simulink model "PMSM_Trapezoidal_ToolBoxST"  (R2013b)
settings: Solver=FixedStepDiscrete  StartTime=0.0  StopTime=10.0  FixedStep=1/5000  RelTol=1e-3
libraries: GPIO_Lib x7, ADC_Lib x3, simulink x3, TIMERS_Lib x1
settings Model: SimulationMode=accelerator  Creator=Alex  LastModifiedBy=reynaudp
settings OptimizationCC: ExpressionDepthLimit=2147483647  OptimizeModelRefInitCode=on  LifeSpan=1
settings DebuggingCC: StateNameClashWarn=warning
settings HardwareCC: ProdLargestAtomicInteger=Integer  ProdLargestAtomicFloat=Float  ProdIntDivRoundTo=Zero  ProdEndianess=LittleEndian  ProdHWDeviceType=STMicroelectronics->STM32F4xx 32-bit Cortex-M4  TargetLargestAtomicInteger=Integer  TargetLargestAtomicFloat=Float  TargetIntDivRoundTo=Zero  TargetEndianess=LittleEndian  TargetHWDeviceType=STMicroelectronics->STM32F4xx 32-bit Cortex-M4
settings RTWCC: SystemTargetFile=stm32F4xx.tlc  TemplateMakefile=stm32F4xx.tmf  Description=stm32F4xx (Embedded Target)  GenerateReport=on  ProcessScript=stm32F4xx_make_rtw_hook  IncludeHyperlinkInReport=on  LaunchReport=on
settings CodeAppCC: IgnoreCustomStorageClasses=off  MaxIdLength=63  CustomSymbolStrType=$N$R$M  InternalIdentifier=Classic
settings STFCustomTargetCC: ParMdlRefBuildCompliant=on  IncludeMdlTerminateFcn=off  CombineOutputUpdateFcns=on  ERTCustomFileBanners=on  SupportContinuousTime=off  SupportNonInlinedSFcns=off  MATLABClassNameForMDSCustomization=Simulink.SoftwareTarget.ERTCustomization  GRTInterface=off  SystemTargetFile=stm32F4xx.tlc
settings ERTTargetCC: CodeReplacementLibrary=ANSI_C  CompOptLevelCompliant=off  ConcurrentExecutionCompliant=off  IncludeMdlTerminateFcn=off  ERTFirstTimeCompliant=off  ModelStepFunctionPrototypeControlCompliant=off  CPPClassGenCompliant=off  InlinedParameterPlacement=NonHierarchical  ERTSrcFileBannerTemplate=sourceFileTemplate.cgt  ERTHdrFileBannerTemplate=sourceFileTemplate.cgt  ERTDataSrcFileTemplate=sourceFileTemplate.cgt  ERTDataHdrFileTemplate=sourceFileTemplate.cgt  ERTCustomFileTemplate=customRoutineProcess.tlc

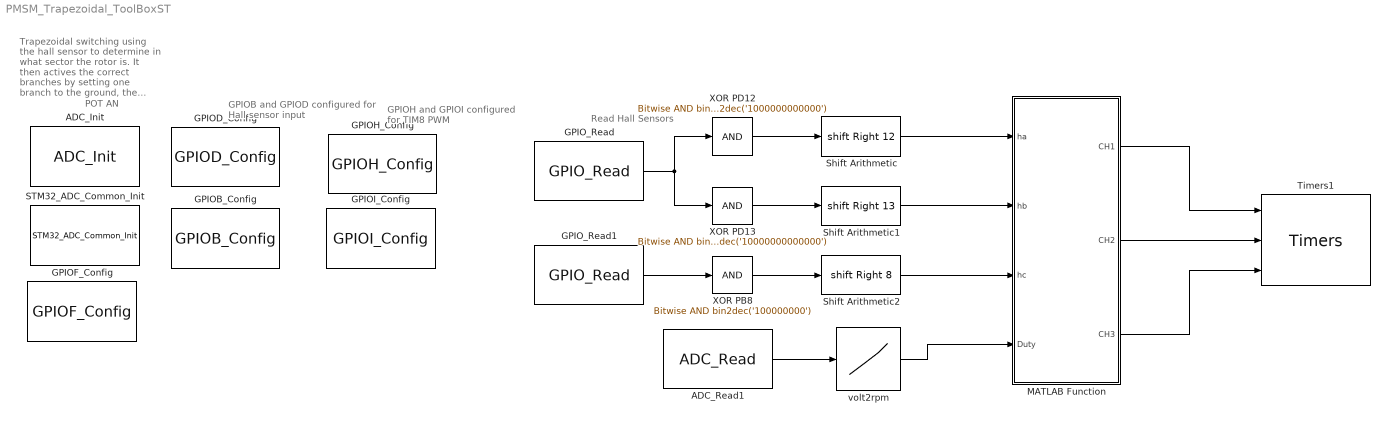
== system PMSM_Trapezoidal_ToolBoxST ==
  note: Trapezoidal switching using the hall sensor to determine in what sector the rotor is. It then actives the correct branches by setting one branch to the ground, the other floating, and the third as PWM pulsing.
      |
      | The PWM duty ratio determines the effective voltage, and thus the speed of the motor. The hall sensors are read using the GPIO, and then the duty is applied to the corresponding PWM channels according to a truth table.
      |
      | Using trapezoidal switching, the current vector is controlled at 30 degree intervals, meaning that the vector is NOT always at 90 degrees with the rotor (which is the optimal control method), but rather oscillates with an error of +- 30 degrees. In this case, a ripple in the torque applied, and the motor produces extra noise, and consumes more current for the same mechanical power output (loss of efficiency)
      |
      | This Algorithm works in open loop (The motor speed is not measured)
  note: POT AN
  note: Read Hall Sensors
  note: GPIOB and GPIOD
      | configured for Hall sensor input
  note: GPIOH and GPIOI
      | configured for TIM8 PWM
  ADC_Init : ADC_Lib/ADC_Init  ADC_Name=ADC3  ADC_Type=Regular  ADC_Default=off  ADC_Offset=0  ADC_Resolution=ADC_Resolution_12b  ADC_ScanConvMode=One_channel  ADC_ContinuousConvMode=on  ADC_ExtTrigPol=ADC_ExternalTrigConvEdge_None  ADC_ExtTrigInjPol=ADC_ExternalTrigInjecConvEdge_None  ADC_ExtTrig=ADC_ExternalTrigConv_T1_CC1  ADC_ExtTrigInj=ADC_ExternalTrigInjecConv_T1_CC4  ADC_DataAlign=ADC_DataAlign_Right  ADC_NbConv=1  ADC_DMA_channel=not_used  ADC_DMA_stream=not_used  ADC_Watchdog_Enable=off  ADC_Watchdog_Command=ADC_AnalogWatchdog_None  ADC_Watchdog_NumChan=0  ADC_Watchdog_HighThreshold=4095  ADC_Watchdog_lowThreshold=0  ADC_Ch0=off  ADC_Ch0T=Regular  ADC_Ch0L=PA0  ADC_Ch1=off  ADC_Ch1T=Regular  ADC_Ch1L=PA1  ADC_Ch2=off  ADC_Ch2T=Regular  ADC_Ch2L=PA2  ADC_Ch3=off  ADC_Ch3T=Regular  ADC_Ch3L=PA3  ADC_Ch4=off  ADC_Ch4T=Regular  ADC_Ch4L=PF6  ADC_Ch5=off  ADC_Ch5T=Regular  ADC_Ch5L=PF7  ADC_Ch6=off  ADC_Ch6T=Regular  ADC_Ch6L=PF8  ADC_Ch7=on  ADC_Ch7T=Regular  ADC_Ch7L=PF9  ADC_Ch8=off  ADC_Ch8T=Regular  ADC_Ch8L=PF10  ADC_Ch9=off  ADC_Ch9T=Regular  ADC_Ch9L=PF3  ADC_Ch10=off  ADC_Ch10T=Regular  ADC_Ch10L=PC0  ADC_Ch11=off  ADC_Ch11T=Regular  ADC_Ch11L=PC1  ADC_Ch12=off  ADC_Ch12T=Regular  ADC_Ch12L=PC2  ADC_Ch13=off  ADC_Ch13T=Regular  ADC_Ch13L=PC3  ADC_Ch14=off  ADC_Ch14T=Regular  ADC_Ch14L=PF4  ADC_Ch15=off  ADC_Ch15T=Regular  ADC_Ch15L=PF5  ADC_Ch16=off  ADC_Ch16T=Regular  ADC_Ch17=off  ADC_Ch17T=Regular  ADC_Ch18=off  ADC_Ch18T=Regular
  ADC_Read1 : ADC_Lib/ADC_Read  ADC_Name=ADC3  ADC_Ch0=off  ADC_Ch1=off  ADC_Ch2=off  ADC_Ch3=off  ADC_Ch4=off  ADC_Ch5=off  ADC_Ch6=off  ADC_Ch7=on  ADC_Ch8=off  ADC_Ch9=off  ADC_Ch10=off  ADC_Ch11=off  ADC_Ch12=off  ADC_Ch13=off  ADC_Ch14=off  ADC_Ch15=off  ADC_Ch16=off  ADC_Ch17=off  ADC_Ch18=off
  GPIOB_Config : GPIO_Lib/GPIOB_Config  Pin0_Use=off  Pin1_Use=off  Pin2_Use=off  Pin3_Use=off  Pin4_Use=off  Pin5_Use=off  Pin6_Use=off  Pin7_Use=off  Pin8_Use=on  Pin9_Use=off  Pin10_Use=off  Pin11_Use=off  Pin12_Use=off  Pin13_Use=off  Pin14_Use=off  Pin15_Use=off  Pin0_Speed=GPIO_Speed_2MHz  Pin1_Speed=GPIO_Speed_2MHz  Pin2_Speed=GPIO_Speed_2MHz  Pin3_Speed=GPIO_Speed_2MHz  Pin4_Speed=GPIO_Speed_2MHz  Pin5_Speed=GPIO_Speed_2MHz  Pin6_Speed=GPIO_Speed_2MHz  Pin7_Speed=GPIO_Speed_2MHz  Pin8_Speed=GPIO_Speed_50MHz  Pin9_Speed=GPIO_Speed_2MHz  Pin10_Speed=GPIO_Speed_2MHz  Pin11_Speed=GPIO_Speed_2MHz  Pin12_Speed=GPIO_Speed_2MHz  Pin13_Speed=GPIO_Speed_2MHz  Pin14_Speed=GPIO_Speed_2MHz  Pin15_Speed=GPIO_Speed_2MHz  Pin0_Mode=GPIO_Mode_OUT  Pin1_Mode=GPIO_Mode_OUT  Pin2_Mode=GPIO_Mode_OUT  Pin3_Mode=GPIO_Mode_OUT  Pin4_Mode=GPIO_Mode_OUT  Pin5_Mode=GPIO_Mode_OUT  Pin6_Mode=GPIO_Mode_OUT  Pin7_Mode=GPIO_Mode_OUT  Pin8_Mode=GPIO_Mode_IN  Pin9_Mode=GPIO_Mode_OUT  Pin10_Mode=GPIO_Mode_OUT  Pin11_Mode=GPIO_Mode_OUT  Pin12_Mode=GPIO_Mode_OUT  Pin13_Mode=GPIO_Mode_OUT  Pin14_Mode=GPIO_Mode_OUT  Pin15_Mode=GPIO_Mode_OUT  Pin0_Type=GPIO_OType_PP  Pin1_Type=GPIO_OType_PP  Pin2_Type=GPIO_OType_PP  Pin3_Type=GPIO_OType_PP  Pin4_Type=GPIO_OType_PP  Pin5_Type=GPIO_OType_PP  Pin6_Type=GPIO_OType_PP  Pin7_Type=GPIO_OType_PP  Pin8_Type=GPIO_OType_PP  Pin9_Type=GPIO_OType_PP  Pin10_Type=GPIO_OType_PP  Pin11_Type=GPIO_OType_PP  Pin12_Type=GPIO_OType_PP  Pin13_Type=GPIO_OType_PP  Pin14_Type=GPIO_OType_PP  Pin15_Type=GPIO_OType_PP  Pin0_PuPd=GPIO_PuPd_NOPULL  Pin1_PuPd=GPIO_PuPd_NOPULL  Pin2_PuPd=GPIO_PuPd_NOPULL  Pin3_PuPd=GPIO_PuPd_NOPULL  Pin4_PuPd=GPIO_PuPd_NOPULL  Pin5_PuPd=GPIO_PuPd_NOPULL  Pin6_PuPd=GPIO_PuPd_NOPULL  Pin7_PuPd=GPIO_PuPd_NOPULL  Pin8_PuPd=GPIO_PuPd_NOPULL  Pin9_PuPd=GPIO_PuPd_NOPULL  Pin10_PuPd=GPIO_PuPd_NOPULL  Pin11_PuPd=GPIO_PuPd_NOPULL  Pin12_PuPd=GPIO_PuPd_NOPULL  Pin13_PuPd=GPIO_PuPd_NOPULL  Pin14_PuPd=GPIO_PuPd_NOPULL  Pin15_PuPd=GPIO_PuPd_NOPULL  Pin0_AF=GPIO_AF_TIM1  Pin1_AF=GPIO_AF_TIM1  Pin3_AF=GPIO_AF_TIM2  Pin4_AF=GPIO_AF_SPI1  Pin5_AF=GPIO_AF_EVENTOUT  Pin6_AF=GPIO_AF_TIM4  Pin7_AF=GPIO_AF_TIM4  Pin8_AF=GPIO_AF_TIM4  Pin9_AF=GPIO_AF_TIM11  Pin10_AF=GPIO_AF_TIM2  Pin11_AF=GPIO_AF_TIM2  Pin12_AF=GPIO_AF_TIM1  Pin13_AF=GPIO_AF_TIM1  Pin14_AF=GPIO_AF_TIM1  Pin15_AF=GPIO_AF_EVENTOUT  Pin0_Set=off  Pin1_Set=off  Pin2_Set=off  Pin3_Set=off  Pin4_Set=off  Pin5_Set=off  Pin6_Set=off  Pin7_Set=off  Pin8_Set=off  Pin9_Set=off  Pin10_Set=off  Pin11_Set=off  Pin12_Set=off  Pin13_Set=off  Pin14_Set=off  Pin15_Set=off
  GPIOD_Config : GPIO_Lib/GPIOD_Config  Pin0_Use=off  Pin1_Use=off  Pin2_Use=off  Pin3_Use=off  Pin4_Use=off  Pin5_Use=off  Pin6_Use=off  Pin7_Use=off  Pin8_Use=off  Pin9_Use=off  Pin10_Use=off  Pin11_Use=off  Pin12_Use=on  Pin13_Use=on  Pin14_Use=off  Pin15_Use=off  Pin0_Speed=GPIO_Speed_2MHz  Pin1_Speed=GPIO_Speed_2MHz  Pin2_Speed=GPIO_Speed_2MHz  Pin3_Speed=GPIO_Speed_2MHz  Pin4_Speed=GPIO_Speed_2MHz  Pin5_Speed=GPIO_Speed_2MHz  Pin6_Speed=GPIO_Speed_2MHz  Pin7_Speed=GPIO_Speed_2MHz  Pin8_Speed=GPIO_Speed_2MHz  Pin9_Speed=GPIO_Speed_2MHz  Pin10_Speed=GPIO_Speed_2MHz  Pin11_Speed=GPIO_Speed_2MHz  Pin12_Speed=GPIO_Speed_100MHz  Pin13_Speed=GPIO_Speed_100MHz  Pin14_Speed=GPIO_Speed_2MHz  Pin15_Speed=GPIO_Speed_2MHz  Pin0_Mode=GPIO_Mode_OUT  Pin1_Mode=GPIO_Mode_OUT  Pin2_Mode=GPIO_Mode_OUT  Pin3_Mode=GPIO_Mode_OUT  Pin4_Mode=GPIO_Mode_OUT  Pin5_Mode=GPIO_Mode_OUT  Pin6_Mode=GPIO_Mode_OUT  Pin7_Mode=GPIO_Mode_OUT  Pin8_Mode=GPIO_Mode_OUT  Pin9_Mode=GPIO_Mode_OUT  Pin10_Mode=GPIO_Mode_OUT  Pin11_Mode=GPIO_Mode_OUT  Pin12_Mode=GPIO_Mode_IN  Pin13_Mode=GPIO_Mode_IN  Pin14_Mode=GPIO_Mode_OUT  Pin15_Mode=GPIO_Mode_OUT  Pin0_Type=GPIO_OType_PP  Pin1_Type=GPIO_OType_PP  Pin2_Type=GPIO_OType_PP  Pin3_Type=GPIO_OType_PP  Pin4_Type=GPIO_OType_PP  Pin5_Type=GPIO_OType_PP  Pin6_Type=GPIO_OType_PP  Pin7_Type=GPIO_OType_PP  Pin8_Type=GPIO_OType_PP  Pin9_Type=GPIO_OType_PP  Pin10_Type=GPIO_OType_PP  Pin11_Type=GPIO_OType_PP  Pin12_Type=GPIO_OType_PP  Pin13_Type=GPIO_OType_PP  Pin14_Type=GPIO_OType_PP  Pin15_Type=GPIO_OType_PP  Pin0_PuPd=GPIO_PuPd_NOPULL  Pin1_PuPd=GPIO_PuPd_NOPULL  Pin2_PuPd=GPIO_PuPd_NOPULL  Pin3_PuPd=GPIO_PuPd_NOPULL  Pin4_PuPd=GPIO_PuPd_NOPULL  Pin5_PuPd=GPIO_PuPd_NOPULL  Pin6_PuPd=GPIO_PuPd_NOPULL  Pin7_PuPd=GPIO_PuPd_NOPULL  Pin8_PuPd=GPIO_PuPd_NOPULL  Pin9_PuPd=GPIO_PuPd_NOPULL  Pin10_PuPd=GPIO_PuPd_NOPULL  Pin11_PuPd=GPIO_PuPd_NOPULL  Pin12_PuPd=GPIO_PuPd_NOPULL  Pin13_PuPd=GPIO_PuPd_NOPULL  Pin14_PuPd=GPIO_PuPd_NOPULL  Pin15_PuPd=GPIO_PuPd_NOPULL  Pin0_AF=GPIO_AF_CAN1  Pin1_AF=GPIO_AF_CAN1  Pin2_AF=GPIO_AF_TIM3  Pin3_AF=GPIO_AF_USART2  Pin4_AF=GPIO_AF_USART2  Pin5_AF=GPIO_AF_EVENTOUT  Pin6_AF=GPIO_AF_USART2  Pin7_AF=GPIO_AF_USART2  Pin8_AF=GPIO_AF_USART3  Pin9_AF=GPIO_AF_USART3  Pin10_AF=GPIO_AF_USART3  Pin11_AF=GPIO_AF_USART3  Pin12_AF=GPIO_AF_TIM4  Pin13_AF=GPIO_AF_TIM4  Pin14_AF=GPIO_AF_TIM4  Pin15_AF=GPIO_AF_EVENTOUT  Pin0_Set=off  Pin1_Set=off  Pin2_Set=off  Pin3_Set=off  Pin4_Set=off  Pin5_Set=off  Pin6_Set=off  Pin7_Set=off  Pin8_Set=off  Pin9_Set=off  Pin10_Set=off  Pin11_Set=off  Pin12_Set=off  Pin13_Set=off  Pin14_Set=off  Pin15_Set=off
  GPIOF_Config : GPIO_Lib/GPIOF_Config  Pin0_Use=off  Pin1_Use=off  Pin2_Use=off  Pin3_Use=off  Pin4_Use=off  Pin5_Use=off  Pin6_Use=off  Pin7_Use=off  Pin8_Use=off  Pin9_Use=on  Pin10_Use=off  Pin11_Use=off  Pin12_Use=off  Pin13_Use=off  Pin14_Use=off  Pin15_Use=off  Pin0_Speed=GPIO_Speed_2MHz  Pin1_Speed=GPIO_Speed_2MHz  Pin2_Speed=GPIO_Speed_2MHz  Pin3_Speed=GPIO_Speed_2MHz  Pin4_Speed=GPIO_Speed_2MHz  Pin5_Speed=GPIO_Speed_2MHz  Pin6_Speed=GPIO_Speed_2MHz  Pin7_Speed=GPIO_Speed_2MHz  Pin8_Speed=GPIO_Speed_2MHz  Pin9_Speed=GPIO_Speed_50MHz  Pin10_Speed=GPIO_Speed_2MHz  Pin11_Speed=GPIO_Speed_2MHz  Pin12_Speed=GPIO_Speed_2MHz  Pin13_Speed=GPIO_Speed_2MHz  Pin14_Speed=GPIO_Speed_2MHz  Pin15_Speed=GPIO_Speed_2MHz  Pin0_Mode=GPIO_Mode_OUT  Pin1_Mode=GPIO_Mode_OUT  Pin2_Mode=GPIO_Mode_OUT  Pin3_Mode=GPIO_Mode_OUT  Pin4_Mode=GPIO_Mode_OUT  Pin5_Mode=GPIO_Mode_OUT  Pin6_Mode=GPIO_Mode_OUT  Pin7_Mode=GPIO_Mode_OUT  Pin8_Mode=GPIO_Mode_OUT  Pin9_Mode=GPIO_Mode_AN  Pin10_Mode=GPIO_Mode_OUT  Pin11_Mode=GPIO_Mode_OUT  Pin12_Mode=GPIO_Mode_OUT  Pin13_Mode=GPIO_Mode_OUT  Pin14_Mode=GPIO_Mode_OUT  Pin15_Mode=GPIO_Mode_OUT  Pin0_Type=GPIO_OType_PP  Pin1_Type=GPIO_OType_PP  Pin2_Type=GPIO_OType_PP  Pin3_Type=GPIO_OType_PP  Pin4_Type=GPIO_OType_PP  Pin5_Type=GPIO_OType_PP  Pin6_Type=GPIO_OType_PP  Pin7_Type=GPIO_OType_PP  Pin8_Type=GPIO_OType_PP  Pin9_Type=GPIO_OType_PP  Pin10_Type=GPIO_OType_PP  Pin11_Type=GPIO_OType_PP  Pin12_Type=GPIO_OType_PP  Pin13_Type=GPIO_OType_PP  Pin14_Type=GPIO_OType_PP  Pin15_Type=GPIO_OType_PP  Pin0_PuPd=GPIO_PuPd_NOPULL  Pin1_PuPd=GPIO_PuPd_NOPULL  Pin2_PuPd=GPIO_PuPd_NOPULL  Pin3_PuPd=GPIO_PuPd_NOPULL  Pin4_PuPd=GPIO_PuPd_NOPULL  Pin5_PuPd=GPIO_PuPd_NOPULL  Pin6_PuPd=GPIO_PuPd_NOPULL  Pin7_PuPd=GPIO_PuPd_NOPULL  Pin8_PuPd=GPIO_PuPd_NOPULL  Pin9_PuPd=GPIO_PuPd_NOPULL  Pin10_PuPd=GPIO_PuPd_NOPULL  Pin11_PuPd=GPIO_PuPd_NOPULL  Pin12_PuPd=GPIO_PuPd_NOPULL  Pin13_PuPd=GPIO_PuPd_NOPULL  Pin14_PuPd=GPIO_PuPd_NOPULL  Pin15_PuPd=GPIO_PuPd_NOPULL  Pin0_AF=GPIO_AF_I2C2  Pin1_AF=GPIO_AF_FSMC  Pin2_AF=GPIO_AF_I2C2  Pin3_AF=GPIO_AF_FSMC  Pin4_AF=GPIO_AF_FSMC  Pin5_AF=GPIO_AF_EVENTOUT  Pin6_AF=GPIO_AF_TIM10  Pin7_AF=GPIO_AF_TIM11  Pin8_AF=GPIO_AF_TIM13  Pin9_AF=GPIO_AF_TIM14  Pin10_AF=GPIO_AF_FSMC  Pin11_AF=GPIO_AF_DCMI  Pin12_AF=GPIO_AF_FSMC  Pin13_AF=GPIO_AF_FSMC  Pin14_AF=GPIO_AF_FSMC  Pin15_AF=GPIO_AF_EVENTOUT  Pin0_Set=off  Pin1_Set=off  Pin2_Set=off  Pin3_Set=off  Pin4_Set=off  Pin5_Set=off  Pin6_Set=off  Pin7_Set=off  Pin8_Set=off  Pin9_Set=off  Pin10_Set=off  Pin11_Set=off  Pin12_Set=off  Pin13_Set=off  Pin14_Set=off  Pin15_Set=off
  GPIOH_Config : GPIO_Lib/GPIOH_Config  Pin0_Use=off  Pin1_Use=off  Pin2_Use=off  Pin3_Use=off  Pin4_Use=off  Pin5_Use=off  Pin6_Use=off  Pin7_Use=off  Pin8_Use=off  Pin9_Use=off  Pin10_Use=off  Pin11_Use=off  Pin12_Use=off  Pin13_Use=on  Pin14_Use=on  Pin15_Use=on  Pin0_Speed=GPIO_Speed_2MHz  Pin1_Speed=GPIO_Speed_2MHz  Pin2_Speed=GPIO_Speed_2MHz  Pin3_Speed=GPIO_Speed_2MHz  Pin4_Speed=GPIO_Speed_2MHz  Pin5_Speed=GPIO_Speed_2MHz  Pin6_Speed=GPIO_Speed_2MHz  Pin7_Speed=GPIO_Speed_2MHz  Pin8_Speed=GPIO_Speed_2MHz  Pin9_Speed=GPIO_Speed_2MHz  Pin10_Speed=GPIO_Speed_2MHz  Pin11_Speed=GPIO_Speed_2MHz  Pin12_Speed=GPIO_Speed_2MHz  Pin13_Speed=GPIO_Speed_2MHz  Pin14_Speed=GPIO_Speed_2MHz  Pin15_Speed=GPIO_Speed_2MHz  Pin0_Mode=GPIO_Mode_OUT  Pin1_Mode=GPIO_Mode_OUT  Pin2_Mode=GPIO_Mode_OUT  Pin3_Mode=GPIO_Mode_OUT  Pin4_Mode=GPIO_Mode_OUT  Pin5_Mode=GPIO_Mode_OUT  Pin6_Mode=GPIO_Mode_OUT  Pin7_Mode=GPIO_Mode_OUT  Pin8_Mode=GPIO_Mode_OUT  Pin9_Mode=GPIO_Mode_OUT  Pin10_Mode=GPIO_Mode_OUT  Pin11_Mode=GPIO_Mode_OUT  Pin12_Mode=GPIO_Mode_OUT  Pin13_Mode=GPIO_Mode_AF  Pin14_Mode=GPIO_Mode_AF  Pin15_Mode=GPIO_Mode_AF  Pin0_Type=GPIO_OType_PP  Pin1_Type=GPIO_OType_PP  Pin2_Type=GPIO_OType_PP  Pin3_Type=GPIO_OType_PP  Pin4_Type=GPIO_OType_PP  Pin5_Type=GPIO_OType_PP  Pin6_Type=GPIO_OType_PP  Pin7_Type=GPIO_OType_PP  Pin8_Type=GPIO_OType_PP  Pin9_Type=GPIO_OType_PP  Pin10_Type=GPIO_OType_PP  Pin11_Type=GPIO_OType_PP  Pin12_Type=GPIO_OType_PP  Pin13_Type=GPIO_OType_PP  Pin14_Type=GPIO_OType_PP  Pin15_Type=GPIO_OType_PP  Pin0_PuPd=GPIO_PuPd_NOPULL  Pin1_PuPd=GPIO_PuPd_NOPULL  Pin2_PuPd=GPIO_PuPd_NOPULL  Pin3_PuPd=GPIO_PuPd_NOPULL  Pin4_PuPd=GPIO_PuPd_NOPULL  Pin5_PuPd=GPIO_PuPd_NOPULL  Pin6_PuPd=GPIO_PuPd_NOPULL  Pin7_PuPd=GPIO_PuPd_NOPULL  Pin8_PuPd=GPIO_PuPd_NOPULL  Pin9_PuPd=GPIO_PuPd_NOPULL  Pin10_PuPd=GPIO_PuPd_NOPULL  Pin11_PuPd=GPIO_PuPd_NOPULL  Pin12_PuPd=GPIO_PuPd_NOPULL  Pin13_PuPd=GPIO_PuPd_NOPULL  Pin14_PuPd=GPIO_PuPd_NOPULL  Pin15_PuPd=GPIO_PuPd_NOPULL  Pin2_AF=GPIO_AF_ETH  Pin3_AF=GPIO_AF_ETH  Pin4_AF=GPIO_AF_I2C2  Pin5_AF=GPIO_AF_EVENTOUT  Pin6_AF=GPIO_AF_I2C2  Pin7_AF=GPIO_AF_I2C3  Pin8_AF=GPIO_AF_I2C3  Pin9_AF=GPIO_AF_I2C3  Pin10_AF=GPIO_AF_TIM5  Pin11_AF=GPIO_AF_TIM5  Pin12_AF=GPIO_AF_TIM5  Pin13_AF=GPIO_AF_TIM8  Pin14_AF=GPIO_AF_TIM8  Pin15_AF=GPIO_AF_TIM8  Pin0_Set=off  Pin1_Set=off  Pin2_Set=off  Pin3_Set=off  Pin4_Set=off  Pin5_Set=off  Pin6_Set=off  Pin7_Set=off  Pin8_Set=off  Pin9_Set=off  Pin10_Set=off  Pin11_Set=off  Pin12_Set=off  Pin13_Set=off  Pin14_Set=off  Pin15_Set=off
  GPIOI_Config : GPIO_Lib/GPIOI_Config  Pin0_Use=off  Pin1_Use=off  Pin2_Use=off  Pin3_Use=off  Pin4_Use=off  Pin5_Use=on  Pin6_Use=on  Pin7_Use=on  Pin8_Use=off  Pin9_Use=off  Pin10_Use=off  Pin11_Use=off  Pin0_Speed=GPIO_Speed_2MHz  Pin1_Speed=GPIO_Speed_2MHz  Pin2_Speed=GPIO_Speed_2MHz  Pin3_Speed=GPIO_Speed_2MHz  Pin4_Speed=GPIO_Speed_2MHz  Pin5_Speed=GPIO_Speed_2MHz  Pin6_Speed=GPIO_Speed_2MHz  Pin7_Speed=GPIO_Speed_2MHz  Pin8_Speed=GPIO_Speed_2MHz  Pin9_Speed=GPIO_Speed_2MHz  Pin10_Speed=GPIO_Speed_2MHz  Pin11_Speed=GPIO_Speed_2MHz  Pin0_Mode=GPIO_Mode_OUT  Pin1_Mode=GPIO_Mode_OUT  Pin2_Mode=GPIO_Mode_OUT  Pin3_Mode=GPIO_Mode_OUT  Pin4_Mode=GPIO_Mode_OUT  Pin5_Mode=GPIO_Mode_AF  Pin6_Mode=GPIO_Mode_AF  Pin7_Mode=GPIO_Mode_AF  Pin8_Mode=GPIO_Mode_OUT  Pin9_Mode=GPIO_Mode_OUT  Pin10_Mode=GPIO_Mode_OUT  Pin11_Mode=GPIO_Mode_OUT  Pin0_Type=GPIO_OType_PP  Pin1_Type=GPIO_OType_PP  Pin2_Type=GPIO_OType_PP  Pin3_Type=GPIO_OType_PP  Pin4_Type=GPIO_OType_PP  Pin5_Type=GPIO_OType_PP  Pin6_Type=GPIO_OType_PP  Pin7_Type=GPIO_OType_PP  Pin8_Type=GPIO_OType_PP  Pin9_Type=GPIO_OType_PP  Pin10_Type=GPIO_OType_PP  Pin11_Type=GPIO_OType_PP  Pin0_PuPd=GPIO_PuPd_NOPULL  Pin1_PuPd=GPIO_PuPd_NOPULL  Pin2_PuPd=GPIO_PuPd_NOPULL  Pin3_PuPd=GPIO_PuPd_NOPULL  Pin4_PuPd=GPIO_PuPd_NOPULL  Pin5_PuPd=GPIO_PuPd_NOPULL  Pin6_PuPd=GPIO_PuPd_NOPULL  Pin7_PuPd=GPIO_PuPd_NOPULL  Pin8_PuPd=GPIO_PuPd_NOPULL  Pin9_PuPd=GPIO_PuPd_NOPULL  Pin10_PuPd=GPIO_PuPd_NOPULL  Pin11_PuPd=GPIO_PuPd_NOPULL  Pin0_AF=GPIO_AF_TIM5  Pin1_AF=GPIO_AF_SPI2  Pin2_AF=GPIO_AF_TIM8  Pin3_AF=GPIO_AF_TIM8  Pin4_AF=GPIO_AF_TIM8  Pin5_AF=GPIO_AF_TIM8  Pin6_AF=GPIO_AF_TIM8  Pin7_AF=GPIO_AF_TIM8  Pin9_AF=GPIO_AF_CAN1  Pin10_AF=GPIO_AF_ETH  Pin11_AF=GPIO_AF_OTG_HS  Pin0_Set=off  Pin1_Set=off  Pin2_Set=off  Pin3_Set=off  Pin4_Set=off  Pin5_Set=off  Pin6_Set=off  Pin7_Set=off  Pin8_Set=off  Pin9_Set=off  Pin10_Set=off  Pin11_Set=off
  GPIO_Read : GPIO_Lib/GPIO_Read  Port_name=GPIOD  Enable_sim=off
  GPIO_Read1 : GPIO_Lib/GPIO_Read  Port_name=GPIOB  Enable_sim=off
  MATLAB Function : MATLAB Function  TreatAsAtomicUnit=on
  STM32_ADC_Common_Init : ADC_Lib/STM32_ADC_Common_Init  ADC_Mode=ADC_Mode_Independent  ADC_Prescaler=ADC_Prescaler_Div2  ADC_DMAAccessMode=ADC_DMAAccessMode_Disabled  ADC_TwoSamplingDelay=ADC_TwoSamplingDelay_5Cycles
  Shift Arithmetic : ArithShift  BitShiftNumber=12  BitShiftDirection=Right
  Shift Arithmetic1 : ArithShift  BitShiftNumber=13  BitShiftDirection=Right
  Shift Arithmetic2 : ArithShift  BitShiftNumber=8  BitShiftDirection=Right
  Timers1 : TIMERS_Lib/Timers  Timer_name=TIM8  Timer_clock=20000000  Timer_mode=TIM_CounterMode_Up  Timer_inout=Output_PWM  Variable_frequency=off  Output_frequency=40000  Encoder_mode=TIM_EncoderMode_TI12  Encoder_auto_reload=0  TRGO_source=not_used  Repetition_counter=0  CH1_enable=on  CH1_type=Output  CH1_int=off  CH1_variable_duty=on  CH1_output_duty=50  CH1_output_polarity=TIM_OCPolarity_Low  CH1_output_comp_state=on  CH1_output_comp_polarity=TIM_OCNPolarity_Low  CH1_output_idle=TIM_OCIdleState_Set  CH1_output_comp_idle=TIM_OCNIdleState_Reset  CH1_input_polarity=TIM_ICPolarity_Rising  CH1_input_prescaler=TIM_ICPSC_DIV1  CH1_input_filter=0  CH1_input_it=No_interrupt  Encoder_TI1_polarity=TIM_ICPolarity_Falling  CH2_enable=on  CH2_type=Output  CH2_int=off  CH2_variable_duty=on  CH2_output_duty=50  CH2_output_polarity=TIM_OCPolarity_Low  CH2_output_comp_state=on  CH2_output_comp_polarity=TIM_OCNPolarity_Low  CH2_output_idle=TIM_OCIdleState_Set  CH2_output_comp_idle=TIM_OCNIdleState_Reset  CH2_input_polarity=TIM_ICPolarity_Rising  CH2_input_prescaler=TIM_ICPSC_DIV1  CH2_input_filter=0  CH2_input_it=No_interrupt  Encoder_TI2_polarity=TIM_ICPolarity_Falling  CH3_enable=on  CH3_type=Output  CH3_int=off  CH3_variable_duty=on  CH3_output_duty=50  CH3_output_polarity=TIM_OCPolarity_Low  CH3_output_comp_state=on  CH3_output_comp_polarity=TIM_OCNPolarity_Low  CH3_output_idle=TIM_OCIdleState_Set  CH3_output_comp_idle=TIM_OCNIdleState_Reset  CH3_input_polarity=TIM_ICPolarity_Rising  CH3_input_prescaler=TIM_ICPSC_DIV1  CH3_input_filter=0  CH3_input_it=No_interrupt
  XOR PB8 : simulink/Logic and Bit Operations/Bitwise Operator  logicop=AND  UseBitMask=on  BitMask=bin2dec('100000000')  BitMaskRealWorld=Stored Integer
  XOR PD12 : simulink/Logic and Bit Operations/Bitwise Operator  logicop=AND  UseBitMask=on  BitMask=bin2dec('1000000000000')  BitMaskRealWorld=Stored Integer
  XOR PD13 : simulink/Logic and Bit Operations/Bitwise Operator  logicop=AND  UseBitMask=on  BitMask=bin2dec('10000000000000')  BitMaskRealWorld=Stored Integer
  volt2rpm : Lookup_n-D  NumberOfTableDimensions=1  BreakpointsForDimension1=[0:100]*(4095/100)  BreakpointsForDimension1Min=0  BreakpointsForDimension1Max=4095  Table=[0:100]  RndMeth=Simplest  InputSameDT=on
  wires:
  GPIO_Read/1 -> XOR PD13/1, XOR PD12/1
  GPIO_Read1/1 -> XOR PB8/1
  XOR PD12/1 -> Shift Arithmetic/1
  XOR PD13/1 -> Shift Arithmetic1/1
  XOR PB8/1 -> Shift Arithmetic2/1
  MATLAB Function/2(CH2) -> Timers1/2
  MATLAB Function/1(CH1) -> Timers1/1
  MATLAB Function/3(CH3) -> Timers1/3
  Shift Arithmetic2/1 -> MATLAB Function/3(hc)
  Shift Arithmetic1/1 -> MATLAB Function/2(hb)
  Shift Arithmetic/1 -> MATLAB Function/1(ha)
  ADC_Read1/1 -> volt2rpm/1
  volt2rpm/1 -> MATLAB Function/4(Duty)

== matlab function PMSM_Trapezoidal_ToolBoxST/MATLAB Function ==
  data: ha input; hb input; hc input; CH1 output; CH2 output; CH3 output; Duty input
function [CH1,CH2,CH3]=Hall_State(ha,hb,hc,Duty)

bc = ha & hb & ~hc;
ba = ~ha & hb & ~hc;
ca = ~ha & hb & hc;
cb = ~ha & ~hb & hc;
ab = ha & ~hb & hc;
ac = ha & ~hb & ~hc;

if bc
    CH1 = (-1);
    CH2 = (Duty);
    CH3 = (0);
elseif ba
    CH1 = (0);
    CH2 = (Duty);
    CH3 = (-1);
elseif ca
    CH1 = (0);
    CH2 = (-1);
    CH3 = (Duty);
elseif cb
    CH1 = (-1);
    CH2 = (0);
    CH3 = (Duty);
elseif ab
    CH1 = (Duty);
    CH2 = (0);
    CH3 = (-1);
elseif ac
    CH1 = (Duty);
    CH2 = (-1);
    CH3 = (0);
else
    CH1 = (-1);
    CH2 = (-1);
    CH3 = (-1);
end
